simulink model "pipeline_state_feedback"  (R2023a)
settings: Solver=ode45  StartTime=0.0  StopTime=200  MaxStep=0.1  RelTol=1e-3
settings Model: Creator=Theodora  LastModifiedBy=Theodora

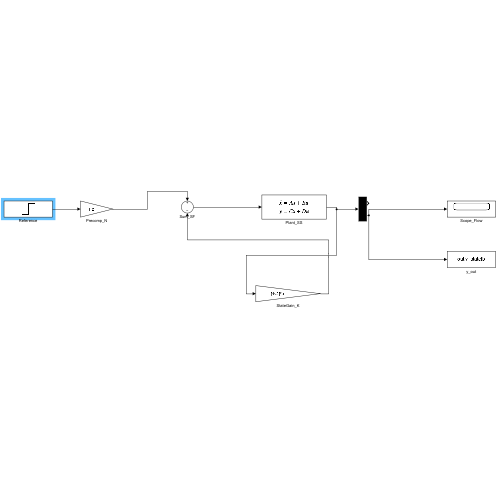
[thumbnail: Simulink's stored preview of the top-level diagram]
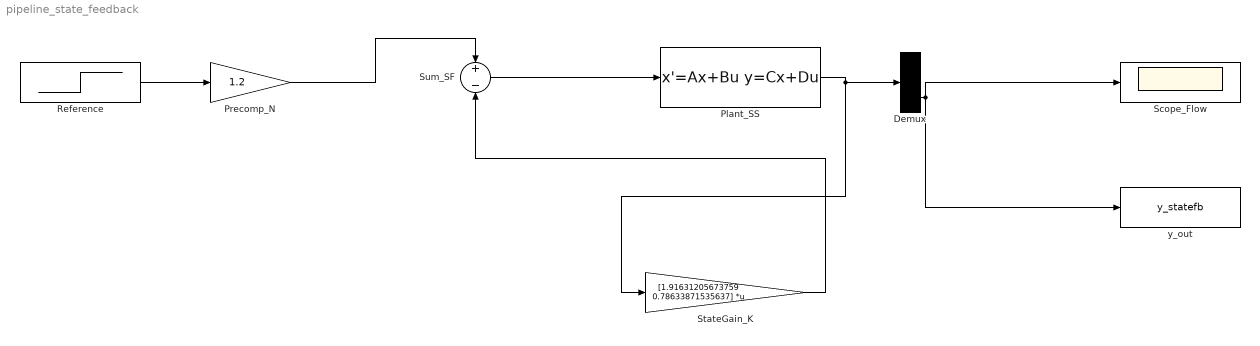
== system pipeline_state_feedback ==
  Demux : Demux  Outputs=2
  Plant_SS : StateSpace  A=[-0.5 0;1 -0.141843971631206]  B=[0.5;0]  C=[1 0;0 1]  D=[0;0]  InitialCondition=[0; 0]
  Precomp_N : Gain  Gain=1.2
  Reference : Step  Time=0  SampleTime=0
  Scope_Flow : Scope
  StateGain_K : Gain  Gain=[1.91631205673759 0.78633871535637]  Multiplication=Matrix(K*u)
  Sum_SF : Sum  Inputs=+-
  y_out : ToWorkspace  VariableName=y_statefb  SampleTime=-1
  wires:
  Reference/1 -> Precomp_N/1
  Precomp_N/1 -> Sum_SF/1
  Sum_SF/1 -> Plant_SS/1
  Plant_SS/1 -> StateGain_K/1, Demux/1
  StateGain_K/1 -> Sum_SF/2
  Demux/2 -> y_out/1, Scope_Flow/1
